simulink model "nh2"  (R2023b)
settings: Solver=ode113  StartTime=0.0  StopTime=10  RelTol=1e-6
values from neighbouring files (symbols this model uses):
  Ic = Iz + 2*Izz + 2*Mk*L^2    (= 6.63214583333)    [dane2nh.m]    (also in danenh.m)
  Ixx = 1/2*Mk*Rkola^2    (= 0.0140625)    [dane2nh.m]    (also in danenh.m)
  k = 1.5    [dane2nh.m]
  Kd = [100,0 ... (first row only)    [dane2nh.m]    (also in danenh.m = [1000,0; lab21.m = [D11,D12)
  L = 0.03    [dane2nh.m]    (also in danenh.m)
  Mc = Mp + 2*Mk    (= 106)    [dane2nh.m]    (also in danenh.m)
  p2 = lambda1+lambda2-k    (= -206.5)    [dane2nh.m]
  p3 = (lambda1*lambda2)/k -p2    (= 7206.5)    [dane2nh.m]
  Rkola = 0.075    [dane2nh.m]    (also in danenh.m)
settings Model: Creator=alozins2  LastModifiedBy=alozins2

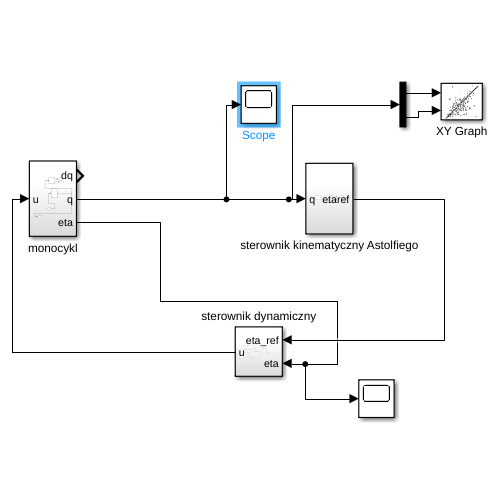
[thumbnail: Simulink's stored preview of the top-level diagram]
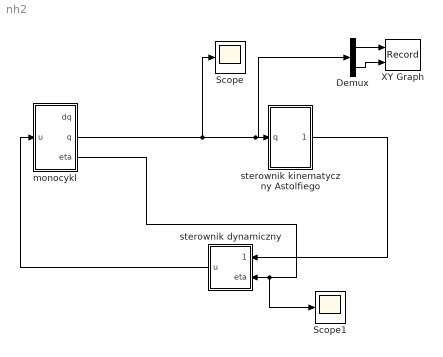
== system nh2 ==
  Demux : Demux  Outputs=2
  Scope : Scope
  Scope1 : Scope
  XY Graph : Record  FileSettingsInternal="{\"entries\":[{\"content\":{\"excelSettings\":{\"content\":{},\"type\":\"Streamout.ExcelSettings\"}},\"type\":\"Streamout.FileSettingStorage\",\"uuid\":\"\"}],\"packageUris\":[\"http:\\/\\/schema.mathworks.com\\/mf0\\/streamout_blocks\\/R2020a\"],\"version\":\"1.0\"}"  Layout=[1 1]  SignalsInternal="{\"entries\":[{\"content\":{\"signals\":[{\"content\":{\"blockPath\":[],\"dimensions\":[2],\"domain\":\"\",\"hasChildren\":true,\"lineColor\":\"#64d413\",\"port\":1,\"sid\":[\"\"],\"signalID\":1,\"signalName\":\"Demux:1\"},\"type\":\"RecordBlkView.Signal\",\"uuid\":\"\"},{\"content\":{\"blockPath\":[],\"channel\":[1],\"dimensions\":[2],\"domain\":\"\",\"lineColor\":\"#7e2f8e\",\"parentID\":1,\"port\":1,\"sid\":[\"\"],\"signalID\":2,\"signalName\":\"Demux:1\"},\"type\":\"RecordBlkView.Signal\",\"uuid\":\"\"},{\"content\":{\"blockPath\":[],\"dimensions\":[1],\"domain\":\"\",\"lineColor\":\"#139fff\",\"plots\":[ 1 ],\"port\":2,\"sid\":[\"\"],\"signalID\":3,\"signalName\":\"Demux:2\"},\"type\":\"RecordBlkView.Signal\",\"uuid\":\"\"},{\"content\":{\"blockPath\":[],\"channel\":[2],\"dimensions\":[2],\"domain\":\"\",\"lineColor\":\"#4dbeee\",\"parentID\":1,\"port\":1,\"sid\":[\"\"],\"signalID\":4,\"signalName\":\"Demux:1\"},\"type\":\"RecordBlkView.Signal\",\"uuid\":\"\"}]},\"type\":\"RecordBlkView.InputSignals\",\"uuid\":\"\"}],\"packageUris\":[\"http:\\/\\/schema.mathworks.com\\/mf0\\/streamout_blocks\\/R2020a\"],\"version\":\"1.0\"}"  VisualizationBindings="{\"xyplotplugin\":{\"info\":[{\"series\":[{\"bindingParametersList\":[{\"parameter\":\"Y-Axis\",\"signalID\":3,\"signalName\":\"Demux:2\"}],\"seriesID\":0}],\"subplotID\":1}]}}"  CompatibilityTag=XY
  monocykl : Subsystem
  sterownik dynamiczny : Subsystem
  sterownik kinematyczny Astolfiego : Subsystem
  wires:
  sterownik dynamiczny/1(u) -> monocykl/1(u)
  sterownik kinematyczny Astolfiego/1(etaref) -> sterownik dynamiczny/1(eta_ref)
  monocykl/3(eta) -> Scope1/1, sterownik dynamiczny/2(eta)
  monocykl/2(q) -> Scope/1, Demux/1, sterownik kinematyczny Astolfiego/1(q)
  Demux/1 -> XY Graph/1
  Demux/2 -> XY Graph/2

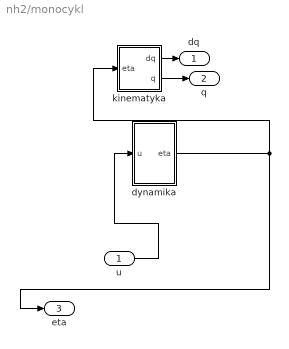
== system nh2/monocykl ==
  u : Inport
  dynamika : Subsystem
  kinematyka : Subsystem
  dq : Outport
  q : Outport  Port=2
  eta : Outport  Port=3
  wires:
  dynamika/1(eta) -> eta/1, kinematyka/1(eta)
  kinematyka/1(dq) -> dq/1
  kinematyka/2(q) -> q/1
  u/1 -> dynamika/1(u)

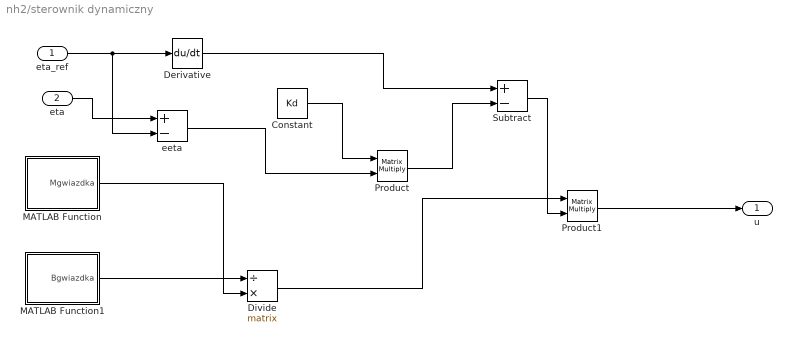
== system nh2/sterownik dynamiczny ==
  eta_ref : Inport
  eta : Inport  Port=2
  Constant : Constant  Value=Kd
  Derivative : Derivative
  Divide : Product  Inputs=/*  Multiplication=Matrix(*)
  MATLAB Function : MATLAB Function  TreatAsAtomicUnit=on
  MATLAB Function1 : MATLAB Function  TreatAsAtomicUnit=on
  Product : Product  Multiplication=Matrix(*)
  Product1 : Product  Multiplication=Matrix(*)
  Subtract : Sum  Inputs=+-
  eeta : Sum  Inputs=+-
  u : Outport
  wires:
  Product1/1 -> u/1
  Constant/1 -> Product/1
  Product/1 -> Subtract/2
  Derivative/1 -> Subtract/1
  MATLAB Function1/1(Bgwiazdka) -> Divide/1
  eta/1 -> eeta/1
  eeta/1 -> Product/2
  Divide/1 -> Product1/1
  MATLAB Function/1(Mgwiazdka) -> Divide/2
  Subtract/1 -> Product1/2
  eta_ref/1 -> eeta/2, Derivative/1

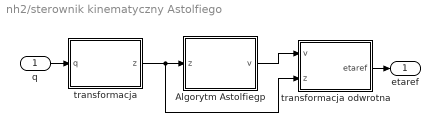
== system nh2/sterownik kinematyczny Astolfiego ==
  q : Inport
  Algorytm Astolfiegp : MATLAB Function  TreatAsAtomicUnit=on
  transformacja : MATLAB Function  TreatAsAtomicUnit=on
  transformacja odwrotna : MATLAB Function  TreatAsAtomicUnit=on
  etaref : Outport
  wires:
  transformacja odwrotna/1(etaref) -> etaref/1
  Algorytm Astolfiegp/1(v) -> transformacja odwrotna/1(v)
  transformacja/1(z) -> transformacja odwrotna/2(z), Algorytm Astolfiegp/1(z)
  q/1 -> transformacja/1(q)

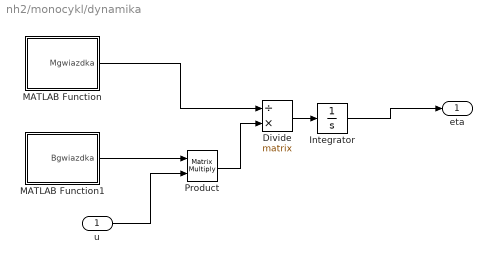
== system nh2/monocykl/dynamika ==
  u : Inport
  Divide : Product  Inputs=/*  Multiplication=Matrix(*)
  Integrator : Integrator  InitialCondition=[0;0]
  MATLAB Function : MATLAB Function  TreatAsAtomicUnit=on
  MATLAB Function1 : MATLAB Function  TreatAsAtomicUnit=on
  Product : Product  Multiplication=Matrix(*)
  eta : Outport
  wires:
  Integrator/1 -> eta/1
  MATLAB Function/1(Mgwiazdka) -> Divide/1
  Product/1 -> Divide/2
  u/1 -> Product/2
  Divide/1 -> Integrator/1
  MATLAB Function1/1(Bgwiazdka) -> Product/1

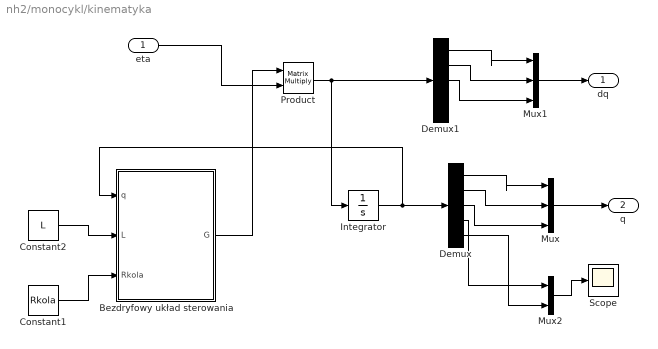
== system nh2/monocykl/kinematyka ==
  eta : Inport
  Bezdryfowy układ sterowania : MATLAB Function  TreatAsAtomicUnit=on
  Constant1 : Constant  Value=Rkola
  Constant2 : Constant  Value=L
  Demux : Demux  Outputs=5
  Demux1 : Demux  Outputs=5
  Integrator : Integrator  InitialCondition=[1;2;pi;0;0]
  Mux : Mux  Inputs=3
  Mux1 : Mux  Inputs=3
  Mux2 : Mux  Inputs=2
  Product : Product  Multiplication=Matrix(*)
  Scope : Scope
  dq : Outport
  q : Outport  Port=2
  wires:
  Integrator/1 -> Demux/1, Bezdryfowy układ sterowania/1(q)
  Product/1 -> Demux1/1, Integrator/1
  Constant1/1 -> Bezdryfowy układ sterowania/3(Rkola)
  Constant2/1 -> Bezdryfowy układ sterowania/2(L)
  eta/1 -> Product/2
  Bezdryfowy układ sterowania/1(G) -> Product/1
  Mux/1 -> q/1
  Demux/1 -> Mux/1
  Demux/2 -> Mux/2
  Demux/3 -> Mux/3
  Demux1/1 -> Mux1/1
  Demux1/3 -> Mux1/3
  Mux1/1 -> dq/1
  Demux1/2 -> Mux1/2
  Demux/4 -> Mux2/1
  Demux/5 -> Mux2/2
  Mux2/1 -> Scope/1

== matlab function nh2/monocykl/kinematyka/Bezdryfowy układ sterowania ==
  data: q input; G output; L input; Rkola input
function G = bezdryfuklster(q,L,Rkola)
teta = q(3);

G = [cos(teta), 0;
    sin(teta),0;
    0,1;
    1/Rkola,L/Rkola;
    1/Rkola, -L/Rkola;];

== matlab function nh2/monocykl/dynamika/MATLAB Function ==
  data: Mc parameter; Ic parameter; Ixx parameter; Rkola parameter; L parameter; Mgwiazdka output
function Mgwiazdka = fcn(Mc, Ic, Ixx, Rkola, L)


Mgwiazdka = [Mc + (2*Ixx)/(Rkola^2), 0;
    0, Ic + (2*Ixx*L^2)/(Rkola^2)];

== matlab function nh2/monocykl/dynamika/MATLAB Function1 ==
  data: Bgwiazdka output; L parameter; Rkola parameter
function Bgwiazdka= fcn(L, Rkola)

Bgwiazdka=[1/Rkola,1/Rkola;
    L/Rkola, -L/Rkola];

== matlab function nh2/sterownik dynamiczny/MATLAB Function ==
  data: Mc parameter; Ic parameter; Ixx parameter; Rkola parameter; L parameter; Mgwiazdka output
function Mgwiazdka = fcn(Mc, Ic, Ixx, Rkola, L)


Mgwiazdka = [Mc + (2*Ixx)/(Rkola^2), 0;
    0, Ic + (2*Ixx*L^2)/(Rkola^2)];

== matlab function nh2/sterownik dynamiczny/MATLAB Function1 ==
  data: Bgwiazdka output; L parameter; Rkola parameter
function Bgwiazdka= fcn(L, Rkola)

Bgwiazdka=[1/Rkola,1/Rkola;
    L/Rkola, -L/Rkola];

== matlab function nh2/sterownik kinematyczny Astolfiego/transformacja ==
  data: q input; z output
function z = T(q)
x=q(1);
y=q(2);
teta=q(3);

z=[teta;
    -x*cos(teta)-y*sin(teta);
    -x*sin(teta)+y*cos(teta)];

== matlab function nh2/sterownik kinematyczny Astolfiego/Algorytm Astolfiegp ==
  data: v output; z input; k parameter; p2 parameter; p3 parameter
function v = Astolf(z, k, p2, p3)

z1=z(1);
z2=z(2);
z3=z(3);

if z1<10^-6
    v=[0;0];
else
v=[-k*z1;
    p2*z2+p3*(z3/z1)];
end

== matlab function nh2/sterownik kinematyczny Astolfiego/transformacja odwrotna ==
  data: v input; etaref output; z input
function etaref = Todwrotne(v,z)

v1=v(1);
v2=v(2);
z3=z(3);

etaref=[v1;
    -v1*z3-v2];
